simulink model "CDCJournalModel"  (R2018b)
settings: Solver=FixedStepAuto  StartTime=0.0  StopTime=p.T  FixedStep=p.Ts  RelTol=1e-3
PreLoadFcn:
  | preLoadCallback
StartFcn:
  | startCallback
StopFcn:
  | stopCallback
values from neighbouring files (symbols this model uses):
  p = simulationParametersClass    [preLoadCallback.m]
  turbineCp = 0.5    [ARPAE30kW_ts.m]
libraries: myLibrary x17, simulink x13, lowLevel x6, controllerComponents x4, performanceIndexComponents x3, headingSetpointCaclulation x1, RLSUpdate_ul x1, dspstat3 x1
(part 1 of 2)
settings Model: PauseTimes=78.131  SnapshotBufferSize=2  SnapshotInterval=1  ExtModeTrigDuration=100  Creator=M.Cobb  LastModifiedBy=mcobb
settings DataIOCC: Decimation=p.decimation  SaveOutput=off  StateSaveName=tmp_raccel_xout  SignalLoggingName=tmp_raccel_logsout
settings OptimizationCC: DefaultParameterBehavior=Inlined  EfficientMapNaN2IntZero=off
settings DebuggingCC: InheritedTsInSrcMsg=none  LibraryContextMissingDiagnostic=none  AllowedUnitSystems=SI,SI (extended)
settings HardwareCC: TargetBitPerPointer=64  TargetBitPerSizeT=64  TargetBitPerPtrDiffT=64  TargetLongLongMode=on  TargetIntDivRoundTo=Zero  TargetEndianess=LittleEndian  TargetWordSize=64  TargetHWDeviceType=MATLAB Host  ProdEqTarget=off
settings SFSimCC: SimUseLocalCustomCode=off
settings RTWCC: SystemTargetFile=raccel.tlc  TemplateMakefile=raccel_default_tmf  RTWVerbose=off  RTWUseLocalCustomCode=off  RTWUseSimCustomCode=on
settings CodeAppCC: GenerateComments=off  MaxIdLength=128  MangleLength=10
settings RaccelTargetCC: GeneratePreprocessorConditionals=Use local settings  MultiInstanceERTCode=off  PreserveStateflowLocalDataDimensions=off  ENABLE_SLEXEC_SSBRIDGE=1  RTWCAPIParams=on

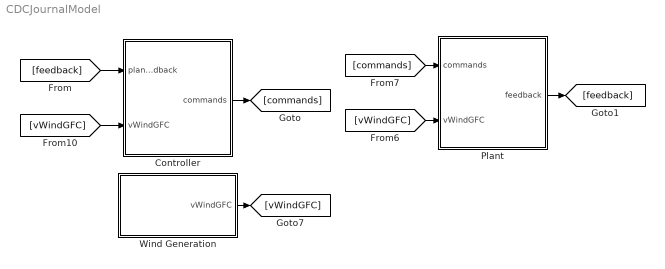
== system CDCJournalModel ==
  Controller : Subsystem  Variant=on
  Plant : Subsystem
  Wind Generation : Subsystem
  wires:
  Wind Generation/1(vWindGFC) -> [vWindGFC]
  [vWindGFC] -> Plant/2(vWindGFC)
  [vWindGFC] -> Controller/2(vWindGFC)
  Controller/1(commands) -> [commands]
  [commands] -> Plant/1(commands)
  Plant/1(feedback) -> [feedback]
  [feedback] -> Controller/1(plantFeedback)

== system CDCJournalModel/Controller ==
  plantFeedback : Inport  OutDataTypeStr=Bus: busPlantFeedback
  vWindGFC : Inport  Port=2
  Optimization Controller : Subsystem  VariantControl=variantControllerOptimization
  Spatial ILC Controller : Subsystem  VariantControl=variantControllerSpatialILC
  commands : Outport  OutDataTypeStr=Bus: busControllerOutput

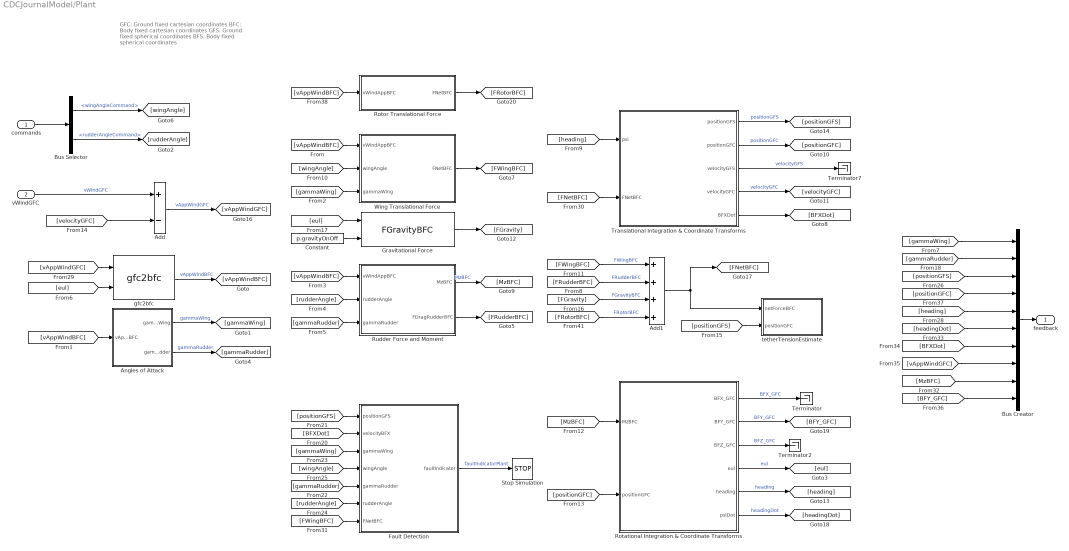
== system CDCJournalModel/Plant ==
  note: GFC: Ground fixed cartesian coordinates
      | BFC:  Body fixed cartesian coordinates
      | GFS: Ground fixed spherical coordinates
      | BFS: Body fixed spherical coordinates
  commands : Inport  OutDataTypeStr=Bus: busControllerOutput
  vWindGFC : Inport  Port=2
  Add : Sum  Inputs=+-
  Add1 : Sum  Inputs=++++
  Angles of Attack : Subsystem
  Bus Selector : BusSelector  OutputSignals=wingAngleCommand,rudderAngleCommand
  Bus Creator : BusCreator  Inputs=10  OutDataTypeStr=Bus: busPlantFeedback
  Constant : Constant  Value=p.gravityOnOff
  Fault Detection : Subsystem
  Gravitational Force : myLibrary/FGravityBFC  SystemSampleTime=-1
  Rotational Integration & Coordinate Transforms : Subsystem
  Rotor Translational Force : Subsystem
  Rudder Force and Moment : Subsystem
  Stop Simulation : Stop
  Terminator : Terminator
  Terminator2 : Terminator
  Terminator7 : Terminator
  Translational Integration & Coordinate Transforms : Subsystem
  Wing Translational Force : Subsystem
  gfc2bfc : myLibrary/gfc2bfc  SystemSampleTime=-1
  tetherTensionEstimate : Subsystem
  feedback : Outport  OutDataTypeStr=Bus: busPlantFeedback
  wires:
  vWindGFC/1 -> Add/1  "vWindGFC"
  [vAppWindBFC] -> Angles of Attack/1(vAppWindBFC)
  Angles of Attack/1(gammaWing) -> [gammaWing]  "gammaWing"
  [vAppWindBFC] -> Wing Translational Force/1(vWindAppBFC)
  Add/1 -> [vAppWindGFC]  "vAppWindGFC"
  [vAppWindBFC] -> Rudder Force and Moment/1(vWindAppBFC)
  [rudderAngle] -> Rudder Force and Moment/2(rudderAngle)
  Translational Integration & Coordinate Transforms/2(positionGFC) -> [positionGFC]  "positionGFC"
  Rudder Force and Moment/2(FDragRudderBFC) -> [FRudderBFC]
  [gammaWing] -> Wing Translational Force/3(gammaWing)
  [heading] -> Translational Integration & Coordinate Transforms/1(psi)
  Angles of Attack/2(gammaRudder) -> [gammaRudder]  "gammaRudder"
  [gammaRudder] -> Rudder Force and Moment/3(gammaRudder)
  Wing Translational Force/1(FNetBFC) -> [FWingBFC]
  [wingAngle] -> Wing Translational Force/2(wingAngle)
  [FNetBFC] -> Translational Integration & Coordinate Transforms/2(FNetBFC)
  Rudder Force and Moment/1(MzBFC) -> [MzBFC]  "MzBFC"
  [MzBFC] -> Rotational Integration & Coordinate Transforms/1(MzBFC)
  [positionGFC] -> Rotational Integration & Coordinate Transforms/2(positionGFC)
  Rotational Integration & Coordinate Transforms/4(eul) -> [eul]  "eul"
  Rotational Integration & Coordinate Transforms/1(BFX_GFC) -> Terminator/1  "BFX_GFC"
  Rotational Integration & Coordinate Transforms/2(BFY_GFC) -> [BFY_GFC]  "BFY_GFC"
  Rotational Integration & Coordinate Transforms/3(BFZ_GFC) -> Terminator2/1  "BFZ_GFC"
  Translational Integration & Coordinate Transforms/4(velocityGFC) -> [velocityGFC]  "velocityGFC"
  [velocityGFC] -> Add/2
  Gravitational Force/1 -> [FGravity]
  [eul] -> Gravitational Force/1
  Translational Integration & Coordinate Transforms/1(positionGFS) -> [positionGFS]  "positionGFS"
  Translational Integration & Coordinate Transforms/3(velocityGFS) -> Terminator7/1  "velocityGFS"
  Rotational Integration & Coordinate Transforms/5(heading) -> [heading]  "heading"
  Constant/1 -> Gravitational Force/2
  Translational Integration & Coordinate Transforms/5(BFXDot) -> [BFXDot]
  [BFXDot] -> Fault Detection/2(velocityBFX)
  [positionGFS] -> Fault Detection/1(positionGFS)
  Fault Detection/1(faultIndicator) -> Stop Simulation/1  "faultIndicatorPlant"
  [gammaRudder] -> Fault Detection/5(gammaRudder)
  [gammaWing] -> Fault Detection/3(gammaWing)
  [rudderAngle] -> Fault Detection/6(rudderAngle)
  [wingAngle] -> Fault Detection/4(wingAngle)
  gfc2bfc/1 -> [vAppWindBFC]  "vAppWindBFC"
  [eul] -> gfc2bfc/2
  [vAppWindGFC] -> gfc2bfc/1
  [FWingBFC] -> Add1/1  "FWingBFC"
  [FGravity] -> Add1/3  "FGravityBFC"
  [FRudderBFC] -> Add1/2  "FRudderBFC"
  Add1/1 -> tetherTensionEstimate/1(netForceBFC), [FNetBFC]
  [FWingBFC] -> Fault Detection/7(FNetBFC)
  commands/1 -> Bus Selector/1
  Bus Selector/1 -> [wingAngle]  "<wingAngleCommand>"
  Bus Selector/2 -> [rudderAngle]  "<rudderAngleCommand>"
  [gammaWing] -> Bus Creator/1
  Bus Creator/1 -> feedback/1
  [gammaRudder] -> Bus Creator/2
  [positionGFS] -> Bus Creator/3
  Rotational Integration & Coordinate Transforms/6(psiDot) -> [headingDot]  "headingDot"
  [BFY_GFC] -> Bus Creator/10
  [MzBFC] -> Bus Creator/9
  [vAppWindGFC] -> Bus Creator/8
  [headingDot] -> Bus Creator/6
  [heading] -> Bus Creator/5
  [BFXDot] -> Bus Creator/7
  [positionGFC] -> Bus Creator/4
  [vAppWindBFC] -> Rotor Translational Force/1(vWindAppBFC)
  Rotor Translational Force/1(FNetBFC) -> [FRotorBFC]
  [FRotorBFC] -> Add1/4  "FRotorBFC"
  [positionGFS] -> tetherTensionEstimate/2(positionGFC)

== system CDCJournalModel/Wind Generation ==
  Constant : Constant  Value=p.windVariant
  Constant Wind : Subsystem
  Constant1 : Constant  Value=[0 0 0]
  Multiport Switch : MultiPortSwitch
  NREL Wind : Subsystem
  vWindGFC : Outport
  wires:
  Multiport Switch/1 -> vWindGFC/1  "vWindGFC"
  Constant Wind/1(vWindGFC) -> [vWindConstant]
  Constant/1 -> Multiport Switch/1
  [vWindConstant] -> Multiport Switch/2
  Constant1/1 -> Multiport Switch/3
  [vWindNREL] -> Multiport Switch/4
  NREL Wind/1(vWindGFC) -> [vWindNREL]

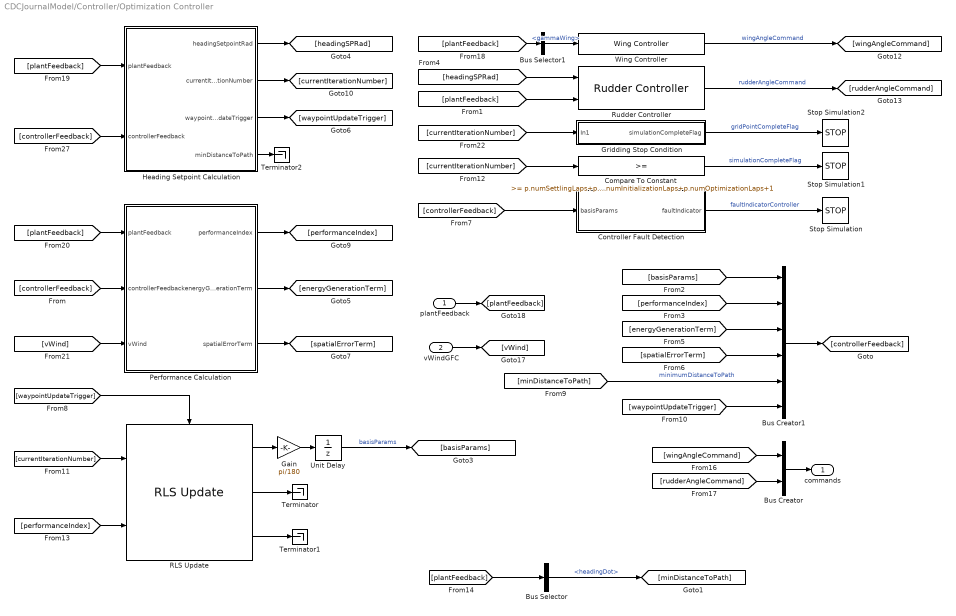
== system CDCJournalModel/Controller/Optimization Controller ==
  plantFeedback : Inport  OutDataTypeStr=Bus: busPlantFeedback
  vWindGFC : Inport  Port=2
  Bus Creator : BusCreator  Inputs=2  OutDataTypeStr=Bus: busControllerOutput
  Bus Creator1 : BusCreator  Inputs=6  OutDataTypeStr=Bus: busControllerFeedback
  Bus Selector : BusSelector  OutputSignals=headingDot
  Bus Selector1 : BusSelector  OutputSignals=gammaWing
  Compare To Constant : simulink/Logic and Bit Operations/Compare To Constant  relop=>=  const=p.numSettlingLaps+p.numInitializationLaps+p.numOptimizationLaps+1  OutDataTypeStr=boolean
  Controller Fault Detection : Subsystem
  Gain : Gain  Gain=pi/180
  Gridding Stop Condition : Subsystem
  Heading Setpoint Calculation : Subsystem  VariantControl=variantPureCarrotFollowing
  Performance Calculation : Subsystem
  RLS Update : RLSUpdate_ul/RLS Update  settlingBasisParameter=[p.width p.height]'  initializationBasisParameters=p.initializationBasisParameters  numSettlingLaps=p.numSettlingLaps  forgettingFactor=p.forgettingFactor  normalizationFactors=p.basisParameterNormalizationFactors'  trustRegionDimensions=p.trustRegionDimensions'  learningGain=p.KLearningGradient  noiseAmplitude=[p.azimuthPerturbationAmplitude p.zenithPerturbationAmplitude]'
  Rudder Controller : controllerComponents/Rudder Controller  SystemSampleTime=-1
  Stop Simulation : Stop
  Stop Simulation1 : Stop
  Stop Simulation2 : Stop
  Terminator : Terminator
  Terminator1 : Terminator
  Terminator2 : Terminator
  Unit Delay : UnitDelay  InitialCondition=[p.width p.height]*pi/180  SampleTime=-1
  Wing Controller : controllerComponents/Wing Controller  SystemSampleTime=-1
  commands : Outport  OutDataTypeStr=Bus: busControllerOutput
  wires:
  Wing Controller/1 -> [wingAngleCommand]  "wingAngleCommand"
  Rudder Controller/1 -> [rudderAngleCommand]  "rudderAngleCommand"
  [headingSPRad] -> Rudder Controller/1
  Controller Fault Detection/1(faultIndicator) -> Stop Simulation/1  "faultIndicatorController"
  Heading Setpoint Calculation/1(headingSetpointRad) -> [headingSPRad]
  Heading Setpoint Calculation/3(waypointUpdateTrigger) -> [waypointUpdateTrigger]
  Heading Setpoint Calculation/2(currentIterationNumber) -> [currentIterationNumber]
  [waypointUpdateTrigger] -> RLS Update/Trigger
  Performance Calculation/1(performanceIndex) -> [performanceIndex]
  [currentIterationNumber] -> RLS Update/1
  Compare To Constant/1 -> Stop Simulation1/1  "simulationCompleteFlag"
  [currentIterationNumber] -> Compare To Constant/1
  [wingAngleCommand] -> Bus Creator/1
  [rudderAngleCommand] -> Bus Creator/2
  Bus Creator/1 -> commands/1
  Bus Selector1/1 -> Wing Controller/1  "<gammaWing>"
  vWindGFC/1 -> [vWind]
  plantFeedback/1 -> [plantFeedback]
  [plantFeedback] -> Bus Selector1/1
  [plantFeedback] -> Performance Calculation/1(plantFeedback)
  [plantFeedback] -> Rudder Controller/2
  [currentIterationNumber] -> Gridding Stop Condition/1(In1)
  Gridding Stop Condition/1(simulationCompleteFlag) -> Stop Simulation2/1  "gridPointCompleteFlag"
  [controllerFeedback] -> Controller Fault Detection/1(basisParams)
  [controllerFeedback] -> Heading Setpoint Calculation/2(controllerFeedback)
  [plantFeedback] -> Heading Setpoint Calculation/1(plantFeedback)
  Heading Setpoint Calculation/4(minDistanceToPath) -> Terminator2/1
  RLS Update/1 -> Gain/1
  [basisParams] -> Bus Creator1/1
  [performanceIndex] -> Bus Creator1/2
  Performance Calculation/2(energyGenerationTerm) -> [energyGenerationTerm]
  Performance Calculation/3(spatialErrorTerm) -> [spatialErrorTerm]
  [energyGenerationTerm] -> Bus Creator1/3
  [spatialErrorTerm] -> Bus Creator1/4
  Bus Creator1/1 -> [controllerFeedback]
  [minDistanceToPath] -> Bus Creator1/5  "minimumDistanceToPath"
  [waypointUpdateTrigger] -> Bus Creator1/6
  [vWind] -> Performance Calculation/3(vWind)
  [controllerFeedback] -> Performance Calculation/2(controllerFeedback)
  Unit Delay/1 -> [basisParams]  "basisParams"
  RLS Update/2 -> Terminator/1
  RLS Update/3 -> Terminator1/1
  Gain/1 -> Unit Delay/1
  [performanceIndex] -> RLS Update/2
  [plantFeedback] -> Bus Selector/1
  Bus Selector/1 -> [minDistanceToPath]  "<headingDot>"

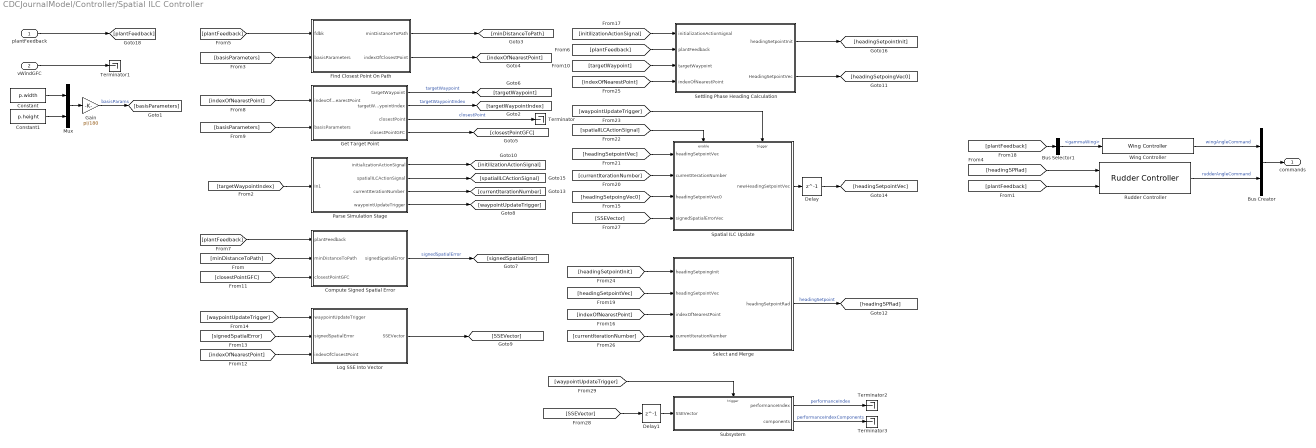
== system CDCJournalModel/Controller/Spatial ILC Controller ==
  plantFeedback : Inport  OutDataTypeStr=Bus: busPlantFeedback
  vWindGFC : Inport  Port=2
  Bus Creator : BusCreator  Inputs=2  OutDataTypeStr=Bus: busControllerOutput
  Bus Selector1 : BusSelector  OutputSignals=gammaWing
  Compute Signed Spatial Error : Subsystem
  Constant : Constant  Value=p.width
  Constant1 : Constant  Value=p.height
  Delay : Delay  DelayLength=1  InitialCondition=0
  Delay1 : Delay  DelayLength=1  InitialCondition=0
  Find Closest Point On Path : Subsystem
  Gain : Gain  Gain=pi/180
  Get Target Point : Subsystem
  Log SSE Into Vector : Subsystem
  Mux : Mux  Inputs=2
  Parse Simulation Stage : Subsystem
  Rudder Controller : controllerComponents/Rudder Controller  SystemSampleTime=-1
  Select and Merge : Subsystem
  Settling Phase Heading Calculation : Subsystem
  Spatial ILC Update : Subsystem
  Subsystem : Subsystem
  Terminator{,1..3} (4 alike) : Terminator
  Wing Controller : controllerComponents/Wing Controller  SystemSampleTime=-1
  commands : Outport  OutDataTypeStr=Bus: busControllerOutput
  wires:
  Wing Controller/1 -> Bus Creator/1  "wingAngleCommand"
  Rudder Controller/1 -> Bus Creator/2  "rudderAngleCommand"
  [headingSPRad] -> Rudder Controller/1
  Bus Creator/1 -> commands/1
  Bus Selector1/1 -> Wing Controller/1  "<gammaWing>"
  vWindGFC/1 -> Terminator1/1
  plantFeedback/1 -> [plantFeedback]
  [plantFeedback] -> Bus Selector1/1
  [plantFeedback] -> Rudder Controller/2
  Get Target Point/3(closestPoint) -> Terminator/1  "closestPoint"
  Find Closest Point On Path/2(indexOfClosestPoint) -> [indexOfNearestPoint]
  [basisParameters] -> Find Closest Point On Path/2(basisParameters)
  Find Closest Point On Path/1(minDistanceToPath) -> [minDistanceToPath]
  Get Target Point/2(targetWaypointIndex) -> [targetWaypointIndex]  "targetWaypointIndex"
  Get Target Point/1(targetWaypoint) -> [targetWaypoint]  "targetWaypoint"
  [indexOfNearestPoint] -> Get Target Point/1(indexOfNearestPoint)
  [basisParameters] -> Get Target Point/2(basisParameters)
  [plantFeedback] -> Find Closest Point On Path/1(fdbk)
  Get Target Point/4(closestPointGFC) -> [closestPointGFC]
  [plantFeedback] -> Compute Signed Spatial Error/1(plantFeedback)
  [minDistanceToPath] -> Compute Signed Spatial Error/2(minDistanceToPath)
  [closestPointGFC] -> Compute Signed Spatial Error/3(closestPointGFC)
  Compute Signed Spatial Error/1(signedSpatialError) -> [signedSpatialError]  "signedSpatialError"
  [waypointUpdateTrigger] -> Log SSE Into Vector/1(waypointUpdateTrigger)
  [signedSpatialError] -> Log SSE Into Vector/2(signedSpatialError)
  [indexOfNearestPoint] -> Log SSE Into Vector/3(indexOfClosestPoint)
  Log SSE Into Vector/1(SSEVector) -> [SSEVector]
  Spatial ILC Update/1(newHeadingSetpointVec) -> Delay/1
  [headingSetpointVec] -> Spatial ILC Update/1(headingSetpointVec)
  [currentIterationNumber] -> Spatial ILC Update/2(currentIterationNumber)
  [headingSetpoingVec0] -> Spatial ILC Update/3(headingSetpointVec0)
  [spatialILCActionSignal] -> Spatial ILC Update/Enable
  [waypointUpdateTrigger] -> Spatial ILC Update/Trigger
  [initilizationActionSignal] -> Settling Phase Heading Calculation/1(initializationActionSignal)
  [plantFeedback] -> Settling Phase Heading Calculation/2(plantFeedback)
  [targetWaypoint] -> Settling Phase Heading Calculation/3(targetWaypoint)
  Settling Phase Heading Calculation/2(HeadingSetpointVec) -> [headingSetpoingVec0]
  [indexOfNearestPoint] -> Select and Merge/3(indexOfNearestPoint)
  Select and Merge/1(headingSetpointRad) -> [headingSPRad]  "headingSetpoint"
  [headingSetpointVec] -> Select and Merge/2(headingSetpointVec)
  Settling Phase Heading Calculation/1(headingSetpointInit) -> [headingSetpointInit]
  [headingSetpointInit] -> Select and Merge/1(headingSetpoingInit)
  [indexOfNearestPoint] -> Settling Phase Heading Calculation/4(indexOfNearestPoint)
  [targetWaypointIndex] -> Parse Simulation Stage/1(In1)
  Parse Simulation Stage/1(initializationActionSignal) -> [initilizationActionSignal]
  Parse Simulation Stage/2(spatialILCActionSignal) -> [spatialILCActionSignal]
  Parse Simulation Stage/3(currentIterationNumber) -> [currentIterationNumber]
  Parse Simulation Stage/4(waypointUpdateTrigger) -> [waypointUpdateTrigger]
  [currentIterationNumber] -> Select and Merge/4(currentIterationNumber)
  Delay/1 -> [headingSetpointVec]
  [SSEVector] -> Spatial ILC Update/4(signedSpatialErrorVec)
  Gain/1 -> [basisParameters]  "basisParams"
  Mux/1 -> Gain/1
  Constant/1 -> Mux/1
  Constant1/1 -> Mux/2
  [SSEVector] -> Delay1/1
  [waypointUpdateTrigger] -> Subsystem/Trigger
  Delay1/1 -> Subsystem/1(SSEVector)
  Subsystem/1(performanceIndex) -> Terminator2/1  "performanceIndex"
  Subsystem/2(components) -> Terminator3/1  "performanceIndexComponents"

== system CDCJournalModel/Plant/Angles of Attack ==
  vAppWindBFC : Inport
  Atan1 : Trigonometry  Operator=atan2
  Atan2 : Trigonometry  Operator=atan2
  Demux : Demux  Outputs=3
  Demux1 : Demux  Outputs=3
  Gain2 : Gain  Gain=-1
  Gain3 : Gain  Gain=-1
  Terminator1 : Terminator
  Terminator2 : Terminator
  deadband : myLibrary/deadband  SystemSampleTime=-1
  deadband1 : myLibrary/deadband  SystemSampleTime=-1
  gammaWing : Outport
  gammaRudder : Outport  Port=2
  wires:
  vAppWindBFC/1 -> Gain2/1
  Demux/1 -> Atan2/2
  Atan2/1 -> Gain3/1
  Atan1/1 -> deadband/1
  Demux/3 -> Atan2/1
  Gain3/1 -> deadband1/1
  Demux/2 -> Terminator1/1
  Demux1/3 -> Terminator2/1
  Gain2/1 -> Demux1/1, Demux/1
  deadband/1 -> gammaRudder/1
  deadband1/1 -> gammaWing/1
  Demux1/1 -> Atan1/2
  Demux1/2 -> Atan1/1

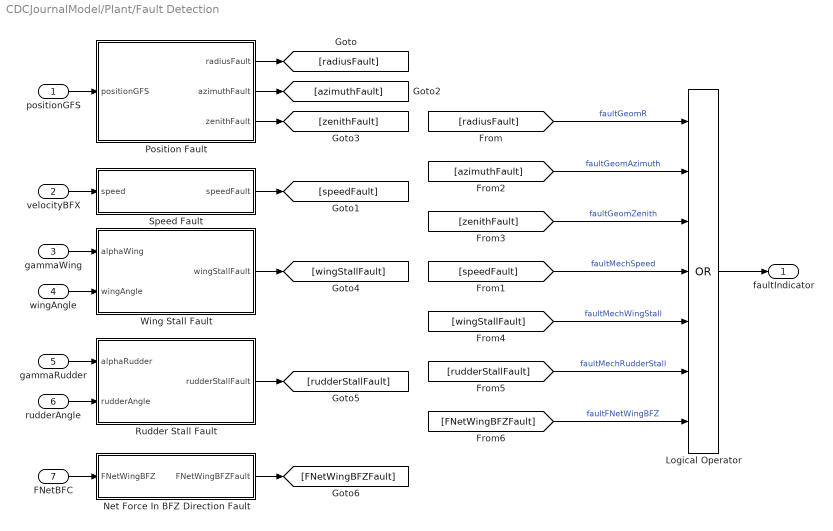
== system CDCJournalModel/Plant/Fault Detection ==
  positionGFS : Inport
  velocityBFX : Inport  Port=2
  gammaWing : Inport  Port=3
  wingAngle : Inport  Port=4
  gammaRudder : Inport  Port=5
  rudderAngle : Inport  Port=6
  FNetBFC : Inport  Port=7
  Logical Operator : Logic  Operator=OR  Inputs=7  AllPortsSameDT=off  OutDataTypeStr=boolean
  Net Force In BFZ Direction Fault : Subsystem
  Position Fault : Subsystem
  Rudder Stall Fault : Subsystem
  Speed Fault : Subsystem
  Wing Stall Fault : Subsystem
  faultIndicator : Outport
  wires:
  positionGFS/1 -> Position Fault/1(positionGFS)
  Logical Operator/1 -> faultIndicator/1
  Speed Fault/1(speedFault) -> [speedFault]
  velocityBFX/1 -> Speed Fault/1(speed)
  [radiusFault] -> Logical Operator/1  "faultGeomR"
  [speedFault] -> Logical Operator/4  "faultMechSpeed"
  [azimuthFault] -> Logical Operator/2  "faultGeomAzimuth"
  [zenithFault] -> Logical Operator/3  "faultGeomZenith"
  Wing Stall Fault/1(wingStallFault) -> [wingStallFault]
  gammaWing/1 -> Wing Stall Fault/1(alphaWing)
  gammaRudder/1 -> Rudder Stall Fault/1(alphaRudder)
  [wingStallFault] -> Logical Operator/5  "faultMechWingStall"
  [rudderStallFault] -> Logical Operator/6  "faultMechRudderStall"
  wingAngle/1 -> Wing Stall Fault/2(wingAngle)
  rudderAngle/1 -> Rudder Stall Fault/2(rudderAngle)
  Rudder Stall Fault/1(rudderStallFault) -> [rudderStallFault]
  Position Fault/1(radiusFault) -> [radiusFault]
  Position Fault/2(azimuthFault) -> [azimuthFault]
  Position Fault/3(zenithFault) -> [zenithFault]
  Net Force In BFZ Direction Fault/1(FNetWingBFZFault) -> [FNetWingBFZFault]
  FNetBFC/1 -> Net Force In BFZ Direction Fault/1(FNetWingBFZ)
  [FNetWingBFZFault] -> Logical Operator/7  "faultFNetWingBFZ"

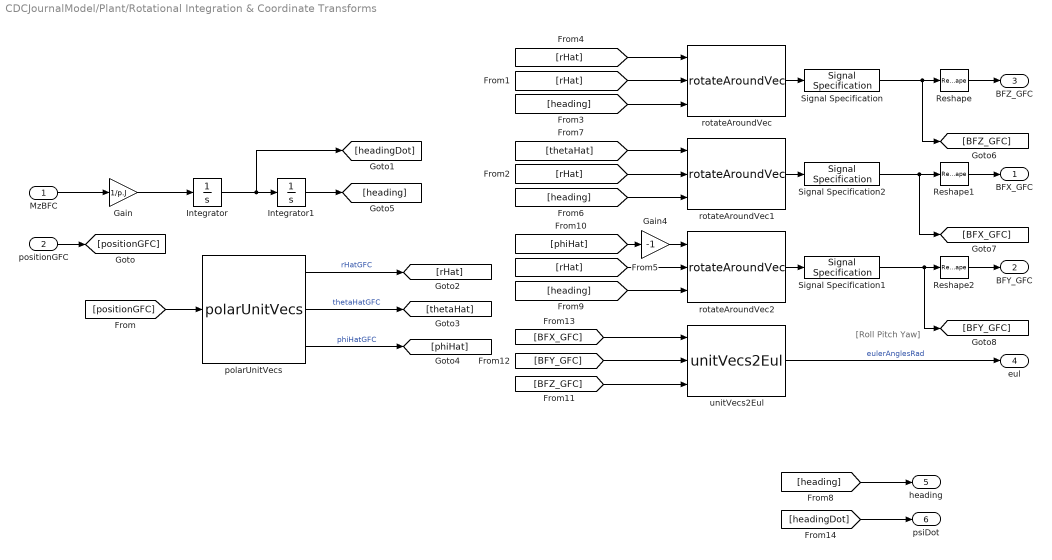
== system CDCJournalModel/Plant/Rotational Integration & Coordinate Transforms ==
  note: [Roll Pitch Yaw]
  MzBFC : Inport  PortDimensions=1
  positionGFC : Inport  Port=2
  Gain : Gain  Gain=1/p.J
  Gain4 : Gain  Gain=-1
  Integrator : Integrator  InitialCondition=p.initOmega
  Integrator1 : Integrator  InitialCondition=p.initTwist
  Reshape : Reshape  OutputDimensions=[3 1]
  Reshape1 : Reshape  OutputDimensions=[3 1]
  Reshape2 : Reshape  OutputDimensions=[3 1]
  Signal Specification : SignalSpecification  Dimensions=[1 3]
  Signal Specification1 : SignalSpecification  Dimensions=[1 3]
  Signal Specification2 : SignalSpecification  Dimensions=[1 3]
  polarUnitVecs : lowLevel/polarUnitVecs  SystemSampleTime=-1
  rotateAroundVec : lowLevel/rotateAroundVec  SystemSampleTime=-1
  rotateAroundVec1 : lowLevel/rotateAroundVec  SystemSampleTime=-1
  rotateAroundVec2 : lowLevel/rotateAroundVec  SystemSampleTime=-1
  unitVecs2Eul : myLibrary/unitVecs2Eul  SystemSampleTime=-1
  BFX_GFC : Outport
  BFY_GFC : Outport  Port=2
  BFZ_GFC : Outport  Port=3
  eul : Outport  Port=4  PortDimensions=3
  heading : Outport  Port=5  PortDimensions=1
  psiDot : Outport  Port=6  PortDimensions=1
  wires:
  MzBFC/1 -> Gain/1
  Integrator/1 -> [headingDot], Integrator1/1
  Gain/1 -> Integrator/1
  positionGFC/1 -> [positionGFC]
  [positionGFC] -> polarUnitVecs/1
  polarUnitVecs/1 -> [rHat]  "rHatGFC"
  polarUnitVecs/2 -> [thetaHat]  "thetaHatGFC"
  polarUnitVecs/3 -> [phiHat]  "phiHatGFC"
  Integrator1/1 -> [heading]
  [heading] -> rotateAroundVec/3
  [rHat] -> rotateAroundVec/1
  [rHat] -> rotateAroundVec/2
  [thetaHat] -> rotateAroundVec1/1
  [heading] -> rotateAroundVec1/3
  [rHat] -> rotateAroundVec1/2
  [phiHat] -> Gain4/1
  [heading] -> rotateAroundVec2/3
  [rHat] -> rotateAroundVec2/2
  unitVecs2Eul/1 -> eul/1  "eulerAnglesRad"
  [BFZ_GFC] -> unitVecs2Eul/3
  [BFY_GFC] -> unitVecs2Eul/2
  [BFX_GFC] -> unitVecs2Eul/1
  Gain4/1 -> rotateAroundVec2/1
  rotateAroundVec/1 -> Signal Specification/1
  rotateAroundVec1/1 -> Signal Specification2/1
  rotateAroundVec2/1 -> Signal Specification1/1
  Signal Specification/1 -> Reshape/1, [BFZ_GFC]
  Signal Specification2/1 -> [BFX_GFC], Reshape1/1
  Signal Specification1/1 -> [BFY_GFC], Reshape2/1
  Reshape/1 -> BFZ_GFC/1
  Reshape1/1 -> BFX_GFC/1
  Reshape2/1 -> BFY_GFC/1
  [heading] -> heading/1
  [headingDot] -> psiDot/1

== system CDCJournalModel/Plant/Rotor Translational Force ==
  vWindAppBFC : Inport
  Constant : Constant  Value=0.5
  Constant1 : Constant  Value=0
  Constant2 : Constant  Value=p.refAreaRotor
  Constant3 : Constant  Value=turbineCp
  Constant4 : Constant  Value=3/2
  Constant5 : Constant  Value=p.numRotors
  Demux1 : Demux  Outputs=3
  Dot Product : DotProduct  InputSameDT=on  OutDataTypeStr=Inherit: Inherit via internal rule
  Gain1 : Gain  Gain=0.5*p.rho*p.refAreaRotor*p.dragCoefficientRotor*p.numRotors
  Multiply : Product  Inputs=5
  Mux1 : Mux  Inputs=3
  Pow : Math  Operator=pow  RndMeth=Zero  SaturateOnIntegerOverflow=on
  Product2 : Product
  Terminator : Terminator
  Terminator1 : Terminator
  normalize1 : myLibrary/normalize  SystemSampleTime=-1
  FNetBFC : Outport
  wires:
  Demux1/3 -> Mux1/3
  Product2/1 -> Demux1/1
  Demux1/1 -> Mux1/1
  Constant1/1 -> Mux1/2
  Demux1/2 -> Terminator1/1
  Mux1/1 -> FNetBFC/1  "FDragRotorBFC"
  vWindAppBFC/1 -> Dot Product/1, normalize1/1, Dot Product/2
  Dot Product/1 -> Pow/1, Gain1/1
  Gain1/1 -> Product2/1  "FDragRotor"
  normalize1/1 -> Product2/2
  Constant/1 -> Multiply/1
  Pow/1 -> Multiply/2
  Constant4/1 -> Pow/2
  Constant3/1 -> Multiply/3
  Constant2/1 -> Multiply/4
  Constant5/1 -> Multiply/5
  Multiply/1 -> Terminator/1  "turbinePower"

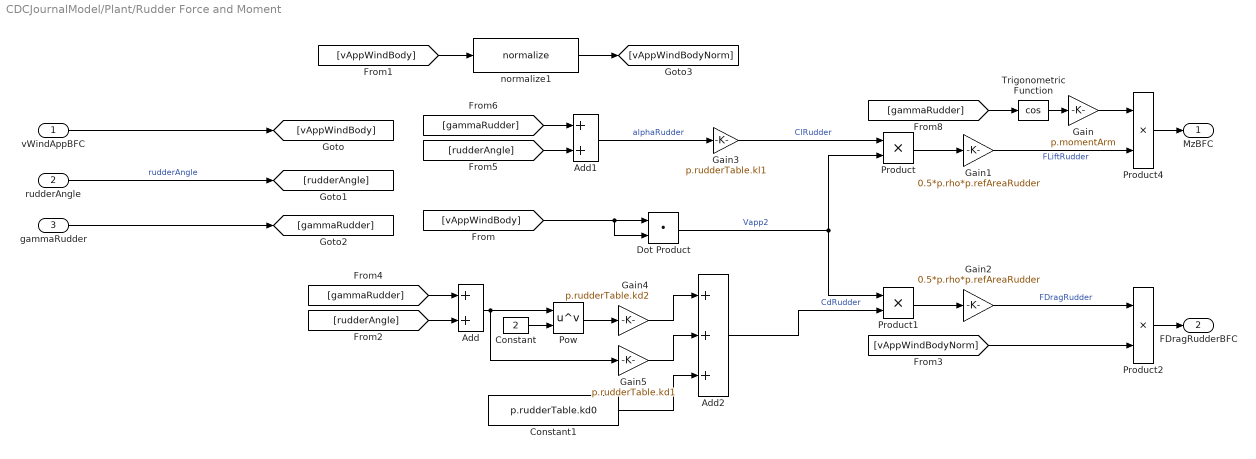
== system CDCJournalModel/Plant/Rudder Force and Moment ==
  vWindAppBFC : Inport
  rudderAngle : Inport  Port=2
  gammaRudder : Inport  Port=3
  Add : Sum
  Add1 : Sum
  Add2 : Sum  Inputs=+++
  Constant : Constant  Value=2
  Constant1 : Constant  Value=p.rudderTable.kd0
  Dot Product : DotProduct  InputSameDT=on  OutDataTypeStr=Inherit: Inherit via internal rule
  Gain : Gain  Gain=p.momentArm
  Gain1 : Gain  Gain=0.5*p.rho*p.refAreaRudder
  Gain2 : Gain  Gain=0.5*p.rho*p.refAreaRudder
  Gain3 : Gain  Gain=p.rudderTable.kl1
  Gain4 : Gain  Gain=p.rudderTable.kd2
  Gain5 : Gain  Gain=p.rudderTable.kd1
  Pow : Math  Operator=pow  RndMeth=Zero  SaturateOnIntegerOverflow=on
  Product{,1..2,4} (4 alike) : Product
  Trigonometric Function : Trigonometry  Operator=cos
  normalize1 : myLibrary/normalize  SystemSampleTime=-1
  MzBFC : Outport
  FDragRudderBFC : Outport  Port=2
  wires:
  Gain3/1 -> Product/1  "ClRudder"
  [vAppWindBody] -> Dot Product/2, Dot Product/1
  Dot Product/1 -> Product1/1, Product/2  "Vapp2"
  vWindAppBFC/1 -> [vAppWindBody]
  Product/1 -> Gain1/1
  Add2/1 -> Product1/2  "CdRudder"
  Product1/1 -> Gain2/1
  Gain2/1 -> Product2/1  "FDragRudder"
  [vAppWindBodyNorm] -> Product2/2
  gammaRudder/1 -> [gammaRudder]
  [rudderAngle] -> Add/2
  [gammaRudder] -> Add/1
  Add/1 -> Gain5/1, Pow/1
  [rudderAngle] -> Add1/2
  [gammaRudder] -> Add1/1
  Add1/1 -> Gain3/1  "alphaRudder"
  Gain1/1 -> Product4/2  "FLiftRudder"
  [vAppWindBody] -> normalize1/1
  normalize1/1 -> [vAppWindBodyNorm]
  Product2/1 -> FDragRudderBFC/1
  [gammaRudder] -> Trigonometric Function/1
  Product4/1 -> MzBFC/1
  Trigonometric Function/1 -> Gain/1
  Gain/1 -> Product4/1
  rudderAngle/1 -> [rudderAngle]  "rudderAngle"
  Constant/1 -> Pow/2
  Pow/1 -> Gain4/1
  Gain4/1 -> Add2/1
  Gain5/1 -> Add2/2
  Constant1/1 -> Add2/3

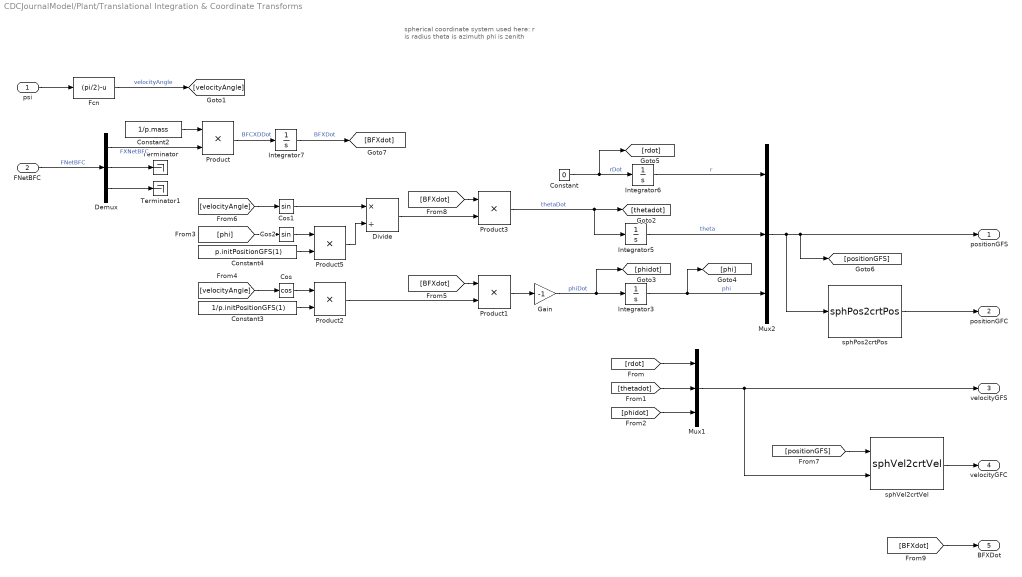
== system CDCJournalModel/Plant/Translational Integration & Coordinate Transforms ==
  note: spherical coordinate system used here:
      | r is radius
      | theta is azimuth
      | phi is zenith
  psi : Inport
  FNetBFC : Inport  Port=2
  Constant : Constant  Value=0
  Constant2 : Constant  Value=1/p.mass
  Constant3 : Constant  Value=1/p.initPositionGFS(1)
  Constant4 : Constant  Value=p.initPositionGFS(1)
  Cos : Trigonometry  Operator=cos
  Cos1 : Trigonometry
  Cos2 : Trigonometry
  Demux : Demux  Outputs=3
  Divide : Product  Inputs=*/
  Fcn : Fcn  Expr=(pi/2)-u
  Gain : Gain  Gain=-1
  Integrator3 : Integrator  InitialCondition=p.initPositionGFS(3)
  Integrator5 : Integrator  InitialCondition=p.initPositionGFS(2)
  Integrator6 : Integrator  InitialCondition=p.initPositionGFS(1)
  Integrator7 : Integrator  InitialCondition=p.initVelocity
  Mux1 : Mux  Inputs=3
  Mux2 : Mux  Inputs=3
  Product{,1..3,5} (5 alike) : Product
  Terminator : Terminator
  Terminator1 : Terminator
  sphPos2crtPos : lowLevel/sphPos2crtPos  SystemSampleTime=-1
  sphVel2crtVel : lowLevel/sphVel2crtVel  SystemSampleTime=-1
  positionGFS : Outport  PortDimensions=3
  positionGFC : Outport  Port=2  PortDimensions=3
  velocityGFS : Outport  Port=3  PortDimensions=3
  velocityGFC : Outport  Port=4  PortDimensions=3
  BFXDot : Outport  Port=5
  wires:
  Gain/1 -> [phidot], Integrator3/1  "phiDot"
  Integrator5/1 -> Mux2/2  "theta"
  Product3/1 -> Integrator5/1, [thetadot]  "thetaDot"
  Integrator3/1 -> [phi], Mux2/3  "phi"
  sphPos2crtPos/1 -> positionGFC/1
  sphVel2crtVel/1 -> velocityGFC/1
  [rdot] -> Mux1/1
  [thetadot] -> Mux1/2
  [phidot] -> Mux1/3
  FNetBFC/1 -> Demux/1  "FNetBFC"
  psi/1 -> Fcn/1
  Demux/1 -> Product/2  "FXNetBFC"
  Integrator6/1 -> Mux2/1  "r"
  Mux1/1 -> sphVel2crtVel/2, velocityGFS/1
  Constant/1 -> [rdot], Integrator6/1  "rDot"
  Mux2/1 -> sphPos2crtPos/1, [positionGFS], positionGFS/1
  [positionGFS] -> sphVel2crtVel/1
  Demux/2 -> Terminator/1
  Demux/3 -> Terminator1/1
  Constant2/1 -> Product/1
  Fcn/1 -> [velocityAngle]  "velocityAngle"
  [BFXdot] -> Product3/1
  [velocityAngle] -> Cos1/1
  Divide/1 -> Product3/2
  Cos1/1 -> Divide/1
  Constant4/1 -> Product5/2
  [phi] -> Cos2/1
  Cos2/1 -> Product5/1
  Product5/1 -> Divide/2
  [BFXdot] -> Product1/1
  [velocityAngle] -> Cos/1
  Product2/1 -> Product1/2
  Cos/1 -> Product2/1
  Constant3/1 -> Product2/2
  Product1/1 -> Gain/1
  Integrator7/1 -> [BFXdot]  "BFXDot"
  Product/1 -> Integrator7/1  "BFCXDDot"
  [BFXdot] -> BFXDot/1

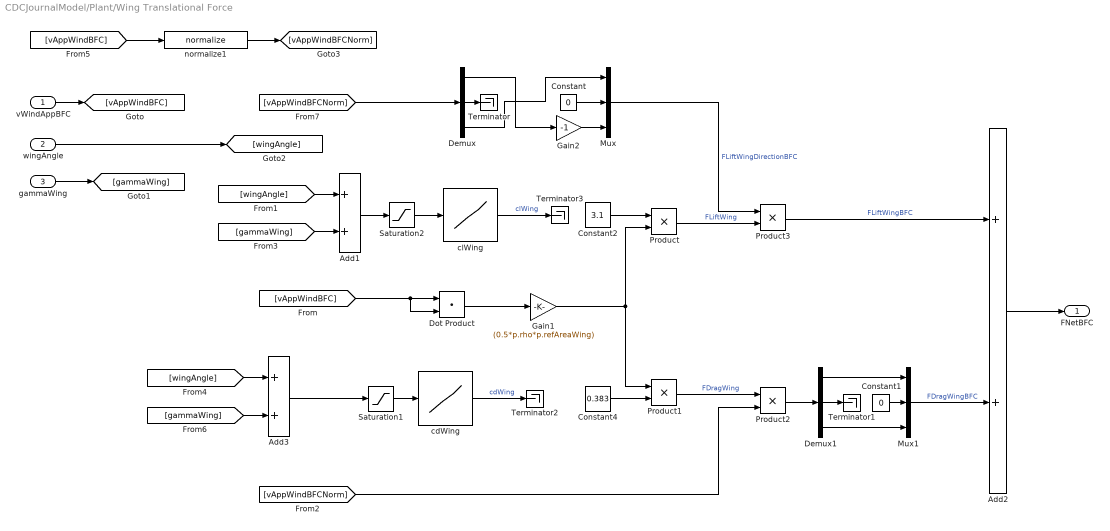
== system CDCJournalModel/Plant/Wing Translational Force ==
  vWindAppBFC : Inport
  wingAngle : Inport  Port=2
  gammaWing : Inport  Port=3
  Add1 : Sum
  Add2 : Sum
  Add3 : Sum
  Constant : Constant  Value=0
  Constant1 : Constant  Value=0
  Constant2 : Constant  Value=3.1
  Constant4 : Constant  Value=0.383
  Demux : Demux  Outputs=3
  Demux1 : Demux  Outputs=3
  Dot Product : DotProduct  InputSameDT=on  OutDataTypeStr=Inherit: Inherit via internal rule
  Gain1 : Gain  Gain=(0.5*p.rho*p.refAreaWing)
  Gain2 : Gain  Gain=-1
  Mux : Mux  Inputs=3
  Mux1 : Mux  Inputs=3
  Product{,1..3} (4 alike) : Product
  Saturation1 : Saturate  UpperLimit=max(p.wingTable.alpha)  LowerLimit=min(p.wingTable.alpha)
  Saturation2 : Saturate  UpperLimit=max(p.wingTable.alpha)  LowerLimit=min(p.wingTable.alpha)
  Terminator{,1..3} (4 alike) : Terminator
  cdWing : Lookup_n-D  NumberOfTableDimensions=1  BreakpointsForDimension1=p.wingTable.alpha  Table=p.wingTable.cd  InternalRulePriority=Speed  RndMeth=Simplest  InputSameDT=on
  clWing : Lookup_n-D  NumberOfTableDimensions=1  BreakpointsForDimension1=p.wingTable.alpha  Table=p.wingTable.cl  InternalRulePriority=Speed  RndMeth=Simplest  InputSameDT=on
  normalize1 : myLibrary/normalize  SystemSampleTime=-1
  FNetBFC : Outport
  wires:
  Product1/1 -> Product2/1  "FDragWing"
  Mux1/1 -> Add2/2  "FDragWingBFC"
  Product/1 -> Product3/2  "FLiftWing"
  Product3/1 -> Add2/1  "FLiftWingBFC"
  Dot Product/1 -> Gain1/1
  clWing/1 -> Terminator3/1  "clWing"
  [vAppWindBFC] -> Dot Product/2, Dot Product/1
  Gain1/1 -> Product/2, Product1/1
  cdWing/1 -> Terminator2/1  "cdWing"
  vWindAppBFC/1 -> [vAppWindBFC]
  Add2/1 -> FNetBFC/1
  gammaWing/1 -> [gammaWing]
  Add3/1 -> Saturation1/1
  [wingAngle] -> Add3/1
  [gammaWing] -> Add3/2
  Demux/2 -> Terminator/1
  Constant/1 -> Mux/2
  Demux/1 -> Gain2/1
  Mux/1 -> Product3/1  "FLiftWingDirectionBFC"
  Demux/3 -> Mux/1
  [vAppWindBFC] -> normalize1/1
  normalize1/1 -> [vAppWindBFCNorm]
  [vAppWindBFCNorm] -> Demux/1
  [vAppWindBFCNorm] -> Product2/2
  Gain2/1 -> Mux/3
  Demux1/2 -> Terminator1/1
  Constant1/1 -> Mux1/2
  Demux1/1 -> Mux1/1
  Product2/1 -> Demux1/1
  Demux1/3 -> Mux1/3
  Saturation1/1 -> cdWing/1
  [wingAngle] -> Add1/1
  [gammaWing] -> Add1/2
  Add1/1 -> Saturation2/1
  wingAngle/1 -> [wingAngle]
  Saturation2/1 -> clWing/1
  Constant2/1 -> Product/1
  Constant4/1 -> Product1/2

== system CDCJournalModel/Plant/tetherTensionEstimate ==
  netForceBFC : Inport
  positionGFC : Inport  Port=2
  Dot Product : DotProduct  InputSameDT=on  OutDataTypeStr=Inherit: Inherit via internal rule
  Multiply : Product
  Selector : Selector  InputPortWidth=3  IndexOptions=Index vector (dialog)  Indices=3  OutputSizes=1
  Sqrt : Sqrt  SaturateOnIntegerOverflow=on
  Terminator : Terminator
  wires:
  positionGFC/1 -> Dot Product/1, Dot Product/2
  Selector/1 -> Multiply/1  "tetherTensionMag"
  Sqrt/1 -> Multiply/2
  netForceBFC/1 -> Selector/1
  Dot Product/1 -> Sqrt/1
  Multiply/1 -> Terminator/1  "tetherTensionVecGFC"

== system CDCJournalModel/Wind Generation/Constant Wind ==
  Constant1 : Constant  Value=0
  Constant4 : Constant  Value=p.vWind
  Mux1 : Mux  Inputs=3
  vWindGFC : Outport
  wires:
  Constant4/1 -> Mux1/1
  Mux1/1 -> vWindGFC/1
  Constant1/1 -> Mux1/2, Mux1/3

== system CDCJournalModel/Wind Generation/NREL Wind ==
  Constant1 : Constant  Value=0
  Constant2 : Constant  Value=p.windDirection
  From Workspace : FromWorkspace  VariableName=windData.NREL  SampleTime=0
  Gain : Gain  Gain=pi/180
  Mux : Mux  Inputs=3
  Product : Product
  Product1 : Product
  Trigonometric Function : Trigonometry
  Trigonometric Function1 : Trigonometry  Operator=cos
  vWindGFC : Outport
  wires:
  Mux/1 -> vWindGFC/1
  Product1/1 -> Mux/2
  Product/1 -> Mux/1
  Trigonometric Function/1 -> Product1/2
  Gain/1 -> Trigonometric Function1/1, Trigonometric Function/1
  Trigonometric Function1/1 -> Product/2
  Constant2/1 -> Gain/1
  Constant1/1 -> Mux/3
  From Workspace/1 -> Product1/1, Product/1

== system CDCJournalModel/Controller/Optimization Controller/Controller Fault Detection ==
  basisParams : Inport  OutDataTypeStr=Bus: busControllerFeedback
  Bus Selector : BusSelector  OutputSignals=basisParams
  Detect Negative Basis Parameters : Subsystem
  faultIndicator : Outport
  wires:
  [faultNegativeBasisParams] -> faultIndicator/1
  Detect Negative Basis Parameters/1(Out1) -> [faultNegativeBasisParams]
  basisParams/1 -> Bus Selector/1
  Bus Selector/1 -> Detect Negative Basis Parameters/1(basisParams)  "<basisParams>"

== system CDCJournalModel/Controller/Optimization Controller/Gridding Stop Condition ==
  In1 : Inport
  Compare To Constant : simulink/Logic and Bit Operations/Compare To Constant  relop===  const=p.numSettlingLaps  OutDataTypeStr=boolean
  Constant : Constant  Value=0
  Constant1 : Constant  Value=p.runModeSwitch
  Multiport Switch : MultiPortSwitch  Inputs=2
  simulationCompleteFlag : Outport
  wires:
  In1/1 -> Compare To Constant/1
  Multiport Switch/1 -> simulationCompleteFlag/1
  Constant/1 -> Multiport Switch/2
  Constant1/1 -> Multiport Switch/1
  Compare To Constant/1 -> Multiport Switch/3

== system CDCJournalModel/Controller/Optimization Controller/Heading Setpoint Calculation ==
  plantFeedback : Inport  OutDataTypeStr=Bus: busPlantFeedback
  controllerFeedback : Inport  Port=2  OutDataTypeStr=Bus: busControllerFeedback
  Bus Selector : BusSelector  OutputSignals=basisParams
  Bus Selector1 : BusSelector  OutputSignals=positionGFS
  Counter : Subsystem
  Detect Iteration Change : Subsystem
  HeadingSetpointCalculation : headingSetpointCaclulation/HeadingSetpointCalculation  searchDistance=p.searchDistance  tol=p.projectionTolerance  meanElev=p.elev  leadLength=p.leadLength  initialPathVariable=p.initialPathVariable
  Terminator : Terminator
  headingSetpointRad : Outport
  currentIterationNumber : Outport  Port=2
  waypointUpdateTrigger : Outport  Port=3
  minDistanceToPath : Outport  Port=4
  wires:
  HeadingSetpointCalculation/1 -> headingSetpointRad/1  "headingSetpoint"
  HeadingSetpointCalculation/4 -> Detect Iteration Change/1(In1)
  Counter/1(Out1) -> currentIterationNumber/1  "currentIterationNumber"
  Detect Iteration Change/1(Out1) -> waypointUpdateTrigger/1, Counter/1(In1)  "waypointUpdateTrigger"
  HeadingSetpointCalculation/2 -> minDistanceToPath/1  "minimumDistanceToPath"
  plantFeedback/1 -> Bus Selector1/1
  controllerFeedback/1 -> Bus Selector/1
  Bus Selector/1 -> HeadingSetpointCalculation/2  "<basisParams>"
  Bus Selector1/1 -> HeadingSetpointCalculation/1  "<positionGFS>"
  HeadingSetpointCalculation/3 -> Terminator/1  "targetPathVariable"

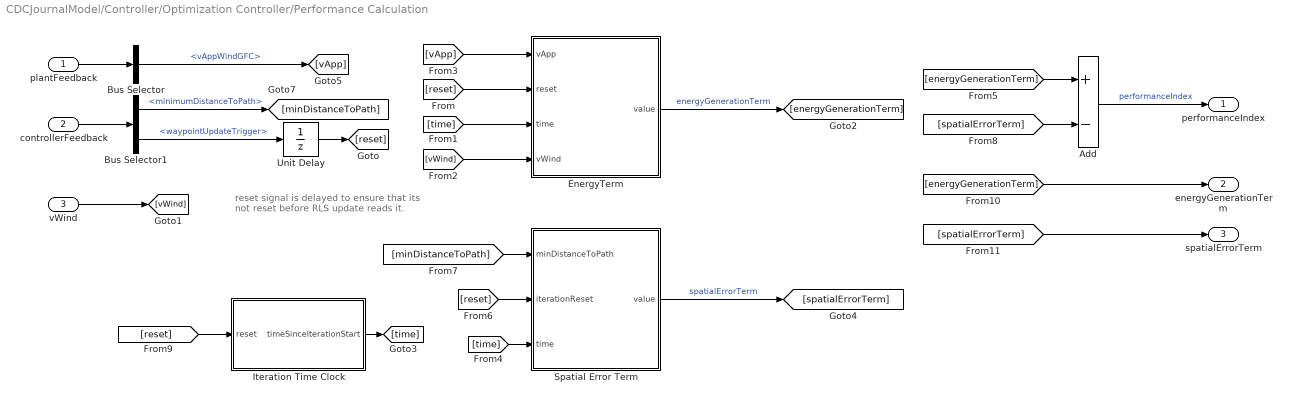
== system CDCJournalModel/Controller/Optimization Controller/Performance Calculation ==
  note: reset signal is delayed to ensure that
      | its not reset before RLS update reads
      | it.
  plantFeedback : Inport  OutDataTypeStr=Bus: busPlantFeedback
  controllerFeedback : Inport  Port=2  OutDataTypeStr=Bus: busControllerFeedback
  vWind : Inport  Port=3
  Add : Sum  Inputs=+-
  Bus Selector : BusSelector  OutputSignals=vAppWindGFC
  Bus Selector1 : BusSelector  OutputSignals=minimumDistanceToPath,waypointUpdateTrigger
  EnergyTerm : Subsystem  Variant=on
  Iteration Time Clock : Subsystem
  Spatial Error Term : Subsystem  Variant=on
  Unit Delay : UnitDelay  InitialCondition=false  SampleTime=-1
  performanceIndex : Outport
  energyGenerationTerm : Outport  Port=2
  spatialErrorTerm : Outport  Port=3
  wires:
  Iteration Time Clock/1(timeSinceIterationStart) -> [time]
  [reset] -> Iteration Time Clock/1(reset)
  Add/1 -> performanceIndex/1  "performanceIndex"
  [reset] -> EnergyTerm/2(reset)
  [time] -> EnergyTerm/3(time)
  [vWind] -> EnergyTerm/4(vWind)
  plantFeedback/1 -> Bus Selector/1
  Bus Selector/1 -> [vApp]  "<vAppWindGFC>"
  [vApp] -> EnergyTerm/1(vApp)
  [time] -> Spatial Error Term/3(time)
  [reset] -> Spatial Error Term/2(iterationReset)
  [minDistanceToPath] -> Spatial Error Term/1(minDistanceToPath)
  EnergyTerm/1(value) -> [energyGenerationTerm]  "energyGenerationTerm"
  Spatial Error Term/1(value) -> [spatialErrorTerm]  "spatialErrorTerm"
  [spatialErrorTerm] -> Add/2
  [energyGenerationTerm] -> Add/1
  [energyGenerationTerm] -> energyGenerationTerm/1
  [spatialErrorTerm] -> spatialErrorTerm/1
  vWind/1 -> [vWind]
  controllerFeedback/1 -> Bus Selector1/1
  Bus Selector1/1 -> [minDistanceToPath]  "<minimumDistanceToPath>"
  Bus Selector1/2 -> Unit Delay/1  "<waypointUpdateTrigger>"
  Unit Delay/1 -> [reset]

== system CDCJournalModel/Controller/Spatial ILC Controller/Compute Signed Spatial Error ==
  plantFeedback : Inport
  minDistanceToPath : Inport  Port=2  Unit=m
  closestPointGFC : Inport  Port=3  Unit=m
  Abs : Abs
  Add : Sum  Inputs=+-
  Bus Selector : BusSelector  OutputSignals=positionGFC,BFY_GFC
  Dot Product : DotProduct  InputSameDT=on  OutDataTypeStr=Inherit: Inherit via internal rule
  Product : Product  Inputs=3
  Sign : Signum
  signedSpatialError : Outport
  wires:
  Add/1 -> Dot Product/1
  closestPointGFC/1 -> Add/1
  Product/1 -> signedSpatialError/1
  Bus Selector/2 -> Dot Product/2  "<BFY_GFC>"
  Dot Product/1 -> Sign/1, Abs/1
  plantFeedback/1 -> Bus Selector/1
  Bus Selector/1 -> Add/2  "<positionGFC>"
  minDistanceToPath/1 -> Product/3
  Abs/1 -> Product/2
  Sign/1 -> Product/1

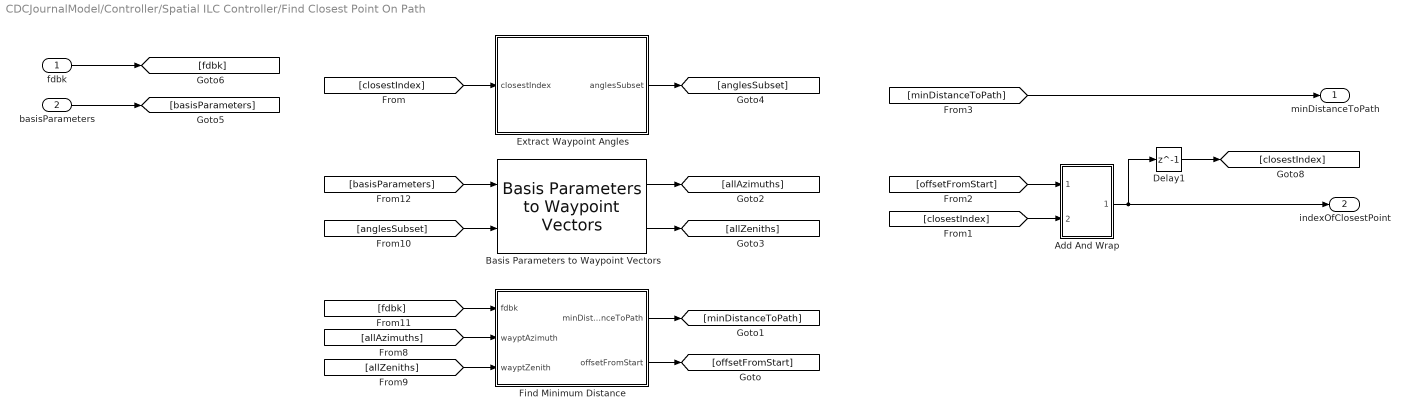
== system CDCJournalModel/Controller/Spatial ILC Controller/Find Closest Point On Path ==
  fdbk : Inport
  basisParameters : Inport  Port=2
  Add And Wrap : Subsystem
  Basis Parameters to Waypoint Vectors : myLibrary/Basis Parameters to Waypoint Vectors
  Delay1 : Delay  DelayLength=1  InitialCondition=1
  Extract Waypoint Angles : Subsystem
  Find Minimum Distance : Subsystem
  minDistanceToPath : Outport
  indexOfClosestPoint : Outport  Port=2
  wires:
  [closestIndex] -> Extract Waypoint Angles/1(closestIndex)
  Basis Parameters to Waypoint Vectors/2 -> [allZeniths]
  Basis Parameters to Waypoint Vectors/1 -> [allAzimuths]
  Extract Waypoint Angles/1(anglesSubset) -> [anglesSubset]
  [anglesSubset] -> Basis Parameters to Waypoint Vectors/2
  basisParameters/1 -> [basisParameters]
  fdbk/1 -> [fdbk]
  [basisParameters] -> Basis Parameters to Waypoint Vectors/1
  [fdbk] -> Find Minimum Distance/1(fdbk)
  [allAzimuths] -> Find Minimum Distance/2(wayptAzimuth)
  [allZeniths] -> Find Minimum Distance/3(wayptZenith)
  Find Minimum Distance/2(offsetFromStart) -> [offsetFromStart]
  [offsetFromStart] -> Add And Wrap/1(offset)
  [closestIndex] -> Add And Wrap/2(startIndex)
  Add And Wrap/1(Out1) -> Delay1/1, indexOfClosestPoint/1
  Delay1/1 -> [closestIndex]
  Find Minimum Distance/1(minDistanceToPath) -> [minDistanceToPath]
  [minDistanceToPath] -> minDistanceToPath/1

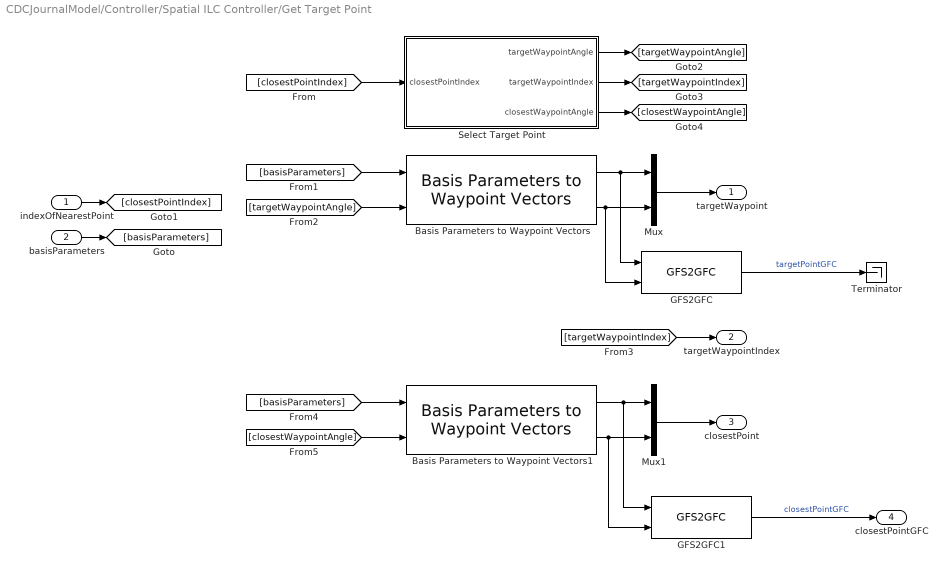
== system CDCJournalModel/Controller/Spatial ILC Controller/Get Target Point ==
  indexOfNearestPoint : Inport
  basisParameters : Inport  Port=2
  Basis Parameters to Waypoint Vectors : myLibrary/Basis Parameters to Waypoint Vectors
  Basis Parameters to Waypoint Vectors1 : myLibrary/Basis Parameters to Waypoint Vectors
  GFS2GFC : myLibrary/GFS2GFC  SystemSampleTime=-1
  GFS2GFC1 : myLibrary/GFS2GFC  SystemSampleTime=-1
  Mux : Mux  Inputs=2
  Mux1 : Mux  Inputs=2
  Select Target Point : Subsystem
  Terminator : Terminator
  targetWaypoint : Outport
  targetWaypointIndex : Outport  Port=2
  closestPoint : Outport  Port=3
  closestPointGFC : Outport  Port=4
  wires:
  Basis Parameters to Waypoint Vectors/1 -> GFS2GFC/1, Mux/1
  Basis Parameters to Waypoint Vectors/2 -> GFS2GFC/2, Mux/2
  basisParameters/1 -> [basisParameters]
  indexOfNearestPoint/1 -> [closestPointIndex]
  [closestPointIndex] -> Select Target Point/1(closestPointIndex)
  [basisParameters] -> Basis Parameters to Waypoint Vectors/1
  Select Target Point/1(targetWaypointAngle) -> [targetWaypointAngle]
  Mux/1 -> targetWaypoint/1
  [targetWaypointAngle] -> Basis Parameters to Waypoint Vectors/2
  Select Target Point/2(targetWaypointIndex) -> [targetWaypointIndex]
  Select Target Point/3(closestWaypointAngle) -> [closestWaypointAngle]
  [targetWaypointIndex] -> targetWaypointIndex/1
  Basis Parameters to Waypoint Vectors1/2 -> GFS2GFC1/2, Mux1/2
  Basis Parameters to Waypoint Vectors1/1 -> GFS2GFC1/1, Mux1/1
  [basisParameters] -> Basis Parameters to Waypoint Vectors1/1
  Mux1/1 -> closestPoint/1
  [closestWaypointAngle] -> Basis Parameters to Waypoint Vectors1/2
  GFS2GFC/1 -> Terminator/1  "targetPointGFC"
  GFS2GFC1/1 -> closestPointGFC/1  "closestPointGFC"

== system CDCJournalModel/Controller/Spatial ILC Controller/Log SSE Into Vector ==
  waypointUpdateTrigger : Inport
  signedSpatialError : Inport  Port=2
  indexOfClosestPoint : Inport  Port=3
  Assignment : Assignment  DiagnosticForDimensions=Warning  IndexOptions=Index vector (port)  Indices=1  OutputSizes=1
  Constant1 : Constant  Value=zeros(p.num,1)
  Delay : Delay  DelayLength=1  InitialCondition=0
  Resettable Delay : Delay  DelayLength=1  InitialConditionSource=Input port  ExternalReset=Rising
      settings: InputPortMap=u0,r5,p4
  SSEVector : Outport
  wires:
  Delay/1 -> Resettable Delay/2
  indexOfClosestPoint/1 -> Assignment/3
  Resettable Delay/1 -> Assignment/1
  signedSpatialError/1 -> Assignment/2
  Assignment/1 -> SSEVector/1, Resettable Delay/1
  waypointUpdateTrigger/1 -> Delay/1
  Constant1/1 -> Resettable Delay/3

== system CDCJournalModel/Controller/Spatial ILC Controller/Parse Simulation Stage ==
  In1 : Inport
  Compare To Constant : simulink/Logic and Bit Operations/Compare To Constant  relop=<=  const=p.numSettlingLaps  OutDataTypeStr=boolean
  Counter : Subsystem
  Detect Iteration Change : Subsystem
  Logical Operator : Logic  Operator=NOT  AllPortsSameDT=off  OutDataTypeStr=boolean
  initializationActionSignal : Outport
  spatialILCActionSignal : Outport  Port=2
  currentIterationNumber : Outport  Port=3
  waypointUpdateTrigger : Outport  Port=4
  wires:
  Counter/1(Out1) -> currentIterationNumber/1, Compare To Constant/1  "currentIterationNumber"
  Detect Iteration Change/1(Out1) -> waypointUpdateTrigger/1, Counter/1(In1)  "waypointUpdateTrigger"
  In1/1 -> Detect Iteration Change/1(In1)
  Logical Operator/1 -> spatialILCActionSignal/1
  Compare To Constant/1 -> Logical Operator/1, initializationActionSignal/1

== system CDCJournalModel/Controller/Spatial ILC Controller/Select and Merge ==
  headingSetpoingInit : Inport
  headingSetpointVec : Inport  Port=2
  indexOfNearestPoint : Inport  Port=3
  currentIterationNumber : Inport  Port=4
  Selector : Selector  InputPortWidth=p.num  IndexOptions=Index vector (port)  Indices=[1 3]  OutputSizes=1
  Switch : Switch  Criteria=u2 > Threshold  Threshold=p.numSettlingLaps
  headingSetpointRad : Outport  Unit=rad
  wires:
  indexOfNearestPoint/1 -> Selector/2
  Switch/1 -> headingSetpointRad/1
  Selector/1 -> Switch/1
  headingSetpointVec/1 -> Selector/1
  headingSetpoingInit/1 -> Switch/3
  currentIterationNumber/1 -> Switch/2

== system CDCJournalModel/Controller/Spatial ILC Controller/Settling Phase Heading Calculation ==
  initializationActionSignal : Inport
  plantFeedback : Inport  Port=2  OutDataTypeStr=Bus: busPlantFeedback
  targetWaypoint : Inport  Port=3  Unit=rad
  indexOfNearestPoint : Inport  Port=4
  Enabled Subsystem1 : Subsystem  TreatAsAtomicUnit=on
  Log Into Vector : Subsystem
  headingSetpointInit : Outport  Unit=rad
  HeadingSetpointVec : Outport  Port=2  Unit=rad
  wires:
  plantFeedback/1 -> Enabled Subsystem1/1(plantFeedback)
  Enabled Subsystem1/1(headingSetpoint) -> Log Into Vector/1(Element), headingSetpointInit/1
  initializationActionSignal/1 -> Enabled Subsystem1/Enable
  targetWaypoint/1 -> Enabled Subsystem1/2(targetWaypoint)
  indexOfNearestPoint/1 -> Log Into Vector/2(Index)
  Log Into Vector/1(headingSetpointVec) -> HeadingSetpointVec/1

== system CDCJournalModel/Controller/Spatial ILC Controller/Spatial ILC Update ==
  headingSetpointVec : Inport  Unit=rad
  currentIterationNumber : Inport  Port=2
  headingSetpointVec0 : Inport  Port=3  Unit=rad
  signedSpatialErrorVec : Inport  Port=4  Unit=m
  Enable : EnablePort
  Trigger : TriggerPort  VariantControl=Variant  PortDimensions=1
  Add : Sum
  Constant2 : Constant  Value=p.spatialILCWeightingMatrix
  Product : Product  Multiplication=Matrix(*)
  Switch : Switch  Criteria=u2 > Threshold  Threshold=p.numSettlingLaps+1
  newHeadingSetpointVec : Outport  Unit=rad
  wires:
  Switch/1 -> Add/1  "spatialILCFirstTerm"
  Product/1 -> Add/2  "spatialILCCorrection"
  headingSetpointVec0/1 -> Switch/3
  currentIterationNumber/1 -> Switch/2
  Constant2/1 -> Product/1
  Add/1 -> newHeadingSetpointVec/1
  headingSetpointVec/1 -> Switch/1
  signedSpatialErrorVec/1 -> Product/2

== system CDCJournalModel/Controller/Spatial ILC Controller/Subsystem ==
  SSEVector : Inport
  Trigger : TriggerPort  VariantControl=Variant  PortDimensions=1
  Abs : Abs
  Constant : Constant  Value=round(p.waypointPathIndices*p.num)
  Selector : Selector  InputPortWidth=p.num  IndexOptions=Index vector (port)  Indices=[1 3]  OutputSizes=1
  Sum of Elements : Sum  Inputs=+
  performanceIndex : Outport
  components : Outport  Port=2
  wires:
  SSEVector/1 -> Selector/1
  Constant/1 -> Selector/2
  Sum of Elements/1 -> performanceIndex/1
  Selector/1 -> Abs/1
  Abs/1 -> components/1, Sum of Elements/1

== system CDCJournalModel/Plant/Fault Detection/Net Force In BFZ Direction Fault ==
  note: If net force in body fixed Z direction is zero or negative
  FNetWingBFZ : Inport
  Compare To Constant : simulink/Logic and Bit Operations/Compare To Constant  relop=<=  const=0  OutDataTypeStr=boolean
  Constant3 : Constant  Value=0
  Demux : Demux  Outputs=3
  Product : Product
  Terminator : Terminator
  Terminator1 : Terminator
  FNetWingBFZFault : Outport
  wires:
  Compare To Constant/1 -> Product/2
  Product/1 -> FNetWingBFZFault/1
  Constant3/1 -> Product/1
  FNetWingBFZ/1 -> Demux/1
  Demux/3 -> Compare To Constant/1  "FNetWingBFZ"
  Demux/1 -> Terminator/1
  Demux/2 -> Terminator1/1

== system CDCJournalModel/Plant/Fault Detection/Position Fault ==
  positionGFS : Inport
  Azimuth Fault : Subsystem
  Constant1 : Constant  Value=0
  Constant2 : Constant
  Constant3 : Constant
  Demux : Demux  Outputs=3
  Product : Product
  Product1 : Product
  Product2 : Product
  Radius Fault : Subsystem
  Zenith Fault : Subsystem
  radiusFault : Outport
  azimuthFault : Outport  Port=2
  zenithFault : Outport  Port=3
  wires:
  positionGFS/1 -> Demux/1
  Demux/1 -> Radius Fault/1(r)
  Radius Fault/1(fault) -> Product2/2
  Azimuth Fault/1(fault) -> Product1/2
  Zenith Fault/1(fault) -> Product/2
  Demux/2 -> Azimuth Fault/1(theta)
  Demux/3 -> Zenith Fault/1(phi)
  Product/1 -> zenithFault/1
  Product1/1 -> azimuthFault/1
  Product2/1 -> radiusFault/1
  Constant3/1 -> Product/1
  Constant1/1 -> Product1/1
  Constant2/1 -> Product2/1

== system CDCJournalModel/Plant/Fault Detection/Rudder Stall Fault ==
  alphaRudder : Inport
  rudderAngle : Inport  Port=2
  Add : Sum
  Compare : RelationalOperator  Operator=<=  OutDataTypeStr=boolean  RndMeth=Nearest  InputSameDT=on
  Compare1 : RelationalOperator  OutDataTypeStr=boolean  RndMeth=Nearest  InputSameDT=on
  Constant : Constant  Value=min(p.rudderTable.alpha)
  Constant1 : Constant  Value=max(p.rudderTable.alpha)
  Constant3 : Constant  Value=0
  Logical Operator : Logic  Operator=OR  AllPortsSameDT=off  OutDataTypeStr=boolean
  Product : Product
  rudderStallFault : Outport
  wires:
  Compare1/1 -> Logical Operator/2
  Constant1/1 -> Compare1/1
  Constant/1 -> Compare/1
  Compare/1 -> Logical Operator/1
  rudderAngle/1 -> Add/2
  alphaRudder/1 -> Add/1
  Add/1 -> Compare1/2, Compare/2
  Constant3/1 -> Product/1
  Logical Operator/1 -> Product/2
  Product/1 -> rudderStallFault/1

== system CDCJournalModel/Plant/Fault Detection/Speed Fault ==
  note: If body fixed speed in x is negative
  speed : Inport
  Compare To Constant : simulink/Logic and Bit Operations/Compare To Constant  relop=<=  const=0  OutDataTypeStr=boolean
  Constant3 : Constant
  Product : Product
  speedFault : Outport
  wires:
  speed/1 -> Compare To Constant/1
  Compare To Constant/1 -> Product/2
  Product/1 -> speedFault/1
  Constant3/1 -> Product/1

== system CDCJournalModel/Plant/Fault Detection/Wing Stall Fault ==
  alphaWing : Inport
  wingAngle : Inport  Port=2
  Add : Sum
  Compare : RelationalOperator  Operator=>  OutDataTypeStr=boolean  RndMeth=Nearest  InputSameDT=on
  Compare1 : RelationalOperator  Operator=<  OutDataTypeStr=boolean  RndMeth=Nearest  InputSameDT=on
  Constant : Constant  Value=min(p.wingTable.alpha)-eps
  Constant1 : Constant  Value=max(p.wingTable.alpha)+eps
  Constant3 : Constant
  Logical Operator : Logic  Operator=OR  AllPortsSameDT=off  OutDataTypeStr=boolean
  Product : Product
  wingStallFault : Outport
  wires:
  Compare/1 -> Logical Operator/1
  Compare1/1 -> Logical Operator/2
  Constant/1 -> Compare/1
  Constant1/1 -> Compare1/1
  alphaWing/1 -> Add/1
  wingAngle/1 -> Add/2
  Add/1 -> Compare1/2, Compare/2
  Logical Operator/1 -> Product/2
  Product/1 -> wingStallFault/1
  Constant3/1 -> Product/1

== system CDCJournalModel/Controller/Optimization Controller/Controller Fault Detection/Detect Negative Basis Parameters ==
  basisParams : Inport
  Compare To Zero : simulink/Logic and Bit Operations/Compare To Zero  relop=<  OutDataTypeStr=boolean
  Compare To Zero1 : simulink/Logic and Bit Operations/Compare To Zero  relop=<  OutDataTypeStr=boolean
  Logical Operator : Logic  Operator=OR  AllPortsSameDT=off  OutDataTypeStr=boolean
  Selector : Selector  InputPortWidth=2  IndexOptions=Index vector (dialog)  Indices=1  OutputSizes=1
  Selector1 : Selector  InputPortWidth=2  IndexOptions=Index vector (dialog)  Indices=1  OutputSizes=1
  Out1 : Outport
  wires:
  Logical Operator/1 -> Out1/1
  Compare To Zero1/1 -> Logical Operator/2  "faultNegativeZenithBasisParam"
  Compare To Zero/1 -> Logical Operator/1  "faultNegativeAzimuthBasisParam"
  basisParams/1 -> Selector/1, Selector1/1
  Selector1/1 -> Compare To Zero1/1
  Selector/1 -> Compare To Zero/1

== system CDCJournalModel/Controller/Optimization Controller/Heading Setpoint Calculation/Counter ==
  In1 : Inport
  Add : Sum
  Data Type Conversion : DataTypeConversion  OutDataTypeStr=uint8
  Memory : Memory  InitialCondition=1
  Out1 : Outport  OutDataTypeStr=double
  wires:
  Add/1 -> Out1/1, Memory/1
  Memory/1 -> Add/2
  In1/1 -> Data Type Conversion/1
  Data Type Conversion/1 -> Add/1
